simulink model "mmerge"  (Simulink 6.3)
settings: Solver=FixedStepDiscrete  StartTime=0.0  StopTime=5  MaxStep=.1  RelTol=1e-3  AbsTol=1e-6
settings Model: Creator=ldean  LastModifiedBy=mshakeri  ExtModeTrigMode=oneshot  ExtModeArmWhenConnect=off  ExtModeAutoUpdateStatusClock=off  StrictBusMsg=ErrorLevel1
settings DataIOCC: LimitDataPoints=off  SaveFormat=StructureWithTime  SaveState=on
settings OptimizationCC: BlockReduction=off  BooleanDataType=off  InlineParams=on  OptimizeModelRefInitCode=on  LifeSpan=1
settings DebuggingCC: SolverPrmCheckMsg=none  IntegerOverflowMsg=none
settings HardwareCC: TargetUnknown=on
settings RTWCC: SystemTargetFile=ert.tlc  TemplateMakefile=ert_default_tmf  RetainRTWFile=on  ProcessScript=ert_make_rtw_hook
settings CodeAppCC: IgnoreCustomStorageClasses=off
settings ERTTargetCC: TargetFcnLib=ansi_tfl_tmw.mat  GenFloatMathFcnCalls=ANSI_C  GenerateSampleERTMain=on  MultiInstanceERTCode=on  InlinedParameterPlacement=NonHierarchical  MultiInstanceErrorCode=None  ERTCustomFileTemplate=example_file_process.tlc  InitialValueSource=Model

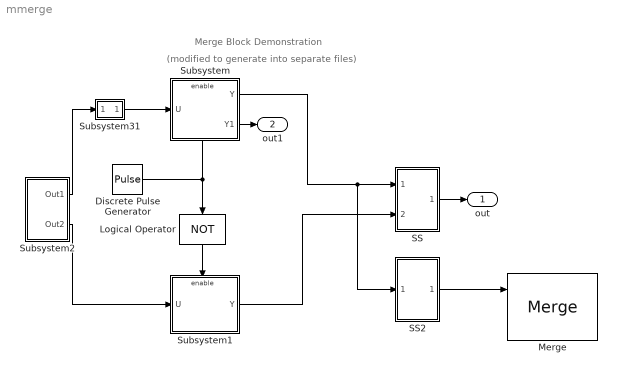
== system mmerge ==
  note: Merge Block Demonstration
  note: (modified to generate into separate files)
  Discrete Pulse Generator : DiscretePulseGenerator  SampleTime=.1
  Logical Operator : Logic  Orientation=down  Operator=NOT  Inputs=1
  Merge : Merge
  SS : Subsystem  TreatAsAtomicUnit=on  RTWFileName=merged
      settings: RTWSystemCode=Function  RTWFileNameOpts=User specified
  SS2 : Subsystem  TreatAsAtomicUnit=on  RTWFileName=merged
      settings: RTWSystemCode=Function  RTWFileNameOpts=User specified
  Subsystem : Subsystem  Tag=MergeExample  TreatAsAtomicUnit=on  RTWFileName=top
      settings: RTWSystemCode=Function  RTWFileNameOpts=User specified
  Subsystem1 : Subsystem  Tag=MergeExample  TreatAsAtomicUnit=on  RTWFileName=bottom
      settings: RTWSystemCode=Function  RTWFileNameOpts=User specified
  Subsystem2 : Subsystem  TreatAsAtomicUnit=on  RTWFileName=source
      settings: RTWSystemCode=Function  RTWFileNameOpts=User specified
  Subsystem31 : Subsystem  mask(clip to zero){threshold=1.0e-6}
      mask Display: disp('clip')
  out : Outport
  out1 : Outport  Port=2
  wires:
  Subsystem2/1(Out1) -> Subsystem31/1(In)
  Subsystem/1(Y) -> SS/1(In1), SS2/1(In1)
  Subsystem1/1(Y) -> SS/2(In2)
  Logical Operator/1 -> Subsystem1/Enable
  Discrete Pulse Generator/1 -> Logical Operator/1, Subsystem/Enable
  Subsystem2/2(Out2) -> Subsystem1/1(U)
  SS/1(out) -> out/1
  Subsystem/2(Y1) -> out1/1
  Subsystem31/1(Out) -> Subsystem/1(U)
  SS2/1(out) -> Merge/1

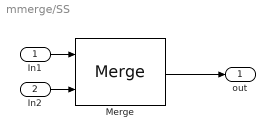
== system mmerge/SS ==
  In1 : Inport  Port=1  LatchInput=off
  In2 : Inport  Port=2  LatchInput=off
  Merge : Merge
  out : Outport
  wires:
  Merge/1 -> out/1
  In1/1 -> Merge/1
  In2/1 -> Merge/2

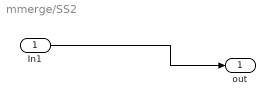
== system mmerge/SS2 ==
  In1 : Inport  Port=1  LatchInput=off
  out : Outport
  wires:
  In1/1 -> out/1

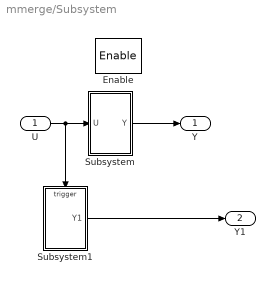
== system mmerge/Subsystem ==
  U : Inport  Port=1  LatchInput=off
  Enable : EnablePort  StatesWhenEnabling=reset  ZeroCross=off
  Subsystem : Subsystem  TreatAsAtomicUnit=on
      settings: RTWSystemCode=Function
  Subsystem1 : Subsystem  TreatAsAtomicUnit=on  RTWFileName=down_counter
      settings: RTWSystemCode=Function  RTWFileNameOpts=User specified
  Y : Outport
  Y1 : Outport  Port=2
  wires:
  Subsystem/1(Y) -> Y/1
  U/1 -> Subsystem/1(U), Subsystem1/Trigger
  Subsystem1/1(Y1) -> Y1/1

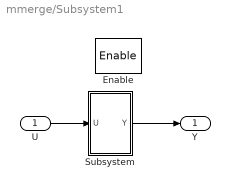
== system mmerge/Subsystem1 ==
  U : Inport  Port=1  LatchInput=off
  Enable : EnablePort  StatesWhenEnabling=reset  ZeroCross=off
  Subsystem : Subsystem  TreatAsAtomicUnit=on
      settings: RTWSystemCode=Function
  Y : Outport
  wires:
  Subsystem/1(Y) -> Y/1
  U/1 -> Subsystem/1(U)

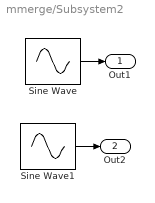
== system mmerge/Subsystem2 ==
  Sine Wave : Sin  Frequency=pi  SampleTime=.1
  Sine Wave1 : Sin  Frequency=pi  Phase=pi  SampleTime=.1
  Out1 : Outport
  Out2 : Outport  Port=2
  wires:
  Sine Wave1/1 -> Out2/1
  Sine Wave/1 -> Out1/1

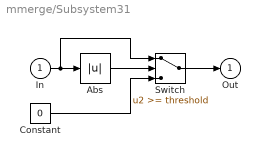
== system mmerge/Subsystem31 ==
  In : Inport  Port=1  LatchInput=off
  Abs : Abs  SaturateOnIntegerOverflow=on
  Constant : Constant  Value=0
  Switch : Switch  Threshold=threshold  SaturateOnIntegerOverflow=on  InputSameDT=on
  Out : Outport  InitialOutput=0
  wires:
  Constant/1 -> Switch/3
  In/1 -> Switch/1, Abs/1
  Switch/1 -> Out/1
  Abs/1 -> Switch/2

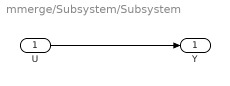
== system mmerge/Subsystem/Subsystem ==
  U : Inport  Port=1  LatchInput=off
  Y : Outport
  wires:
  U/1 -> Y/1

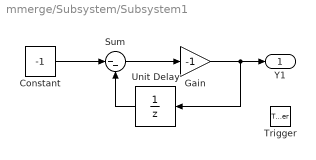
== system mmerge/Subsystem/Subsystem1 ==
  Trigger : TriggerPort  ZeroCross=off
  Constant : Constant  Value=-1
  Gain : Gain  Gain=-1  SaturateOnIntegerOverflow=on
  Sum : Sum  Inputs=|--  SaturateOnIntegerOverflow=on  InputSameDT=on
  Unit Delay : UnitDelay  Orientation=left  SampleTime=-1
  Y1 : Outport
  wires:
  Constant/1 -> Sum/1
  Sum/1 -> Gain/1
  Gain/1 -> Y1/1, Unit Delay/1
  Unit Delay/1 -> Sum/2

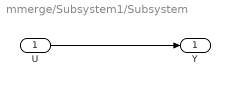
== system mmerge/Subsystem1/Subsystem ==
  U : Inport  Port=1  LatchInput=off
  Y : Outport
  wires:
  U/1 -> Y/1
